simulink model "MMAE_laneChangeParametricWithMeasurements"  (R2018b)
settings: Solver=FixedStepAuto  StartTime=0.0  StopTime=15  FixedStep=1e-3  RelTol=1e-3
values from neighbouring files (symbols this model uses):
  A = obj.A    [LeftLaneChangeRelativeMotionModel.m]    (also in initialization.m = 1.75; laneChangeSinusoidalFcn.m = 1.75; laneChangeSinusoidalJacobianFcn.m = 1.75; leftLaneChangeParametricFcn.m = lateral_dist/2)
  Ts = 0.1    [KinematicBicycleModel.m]    (also in LeftLaneChangeSinusoidalMotionModel.m; LinearizedBicycleModel.m; SimplifiedKinematicBicycleModel.m; amm_rel_test.m)
  vx = X(2)    [cv_model_fun.m]    (also in initialization.m = 10)
  vy = X(4)    [cv_model_fun.m]    (also in initialization.m = 0)
  w = obj.w    [LeftLaneChangeRelativeMotionModel.m]    (also in ctra_model_fun.m = X(6); ctrv_model_fun.m = X(5); initialization.m = 0.0314159265359; laneChangeSinusoidalFcn.m = 0.0209439510239)
  x = X(1)    [KinematicBicycleModel.m]    (also in SimplifiedKinematicBicycleModel.m; behavior_model.m = 0:0.01:20; cca_model_fun.m; ctra_model_fun.m)
  y = X(2)    [KinematicBicycleModel.m]    (also in SimplifiedKinematicBicycleModel.m; behavior_model.m = [distances velocities]; cca_model_fun.m; ctra_model_fun.m)
  y_init = lanewidth/2    (= 1.75)    [initialization.m]    (also in laneChangeSinusoidalFcn.m; laneChangeSinusoidalJacobianFcn.m; leftLaneChangeSinusoidalFcn.m; leftLaneChangeSinusoidalJacobianFcn.m)
libraries: simulink x7
settings Model: Creator=jasprit  LastModifiedBy=jasprit
settings SFSimCC: SimUseLocalCustomCode=off
settings RTWCC: RTWUseLocalCustomCode=off

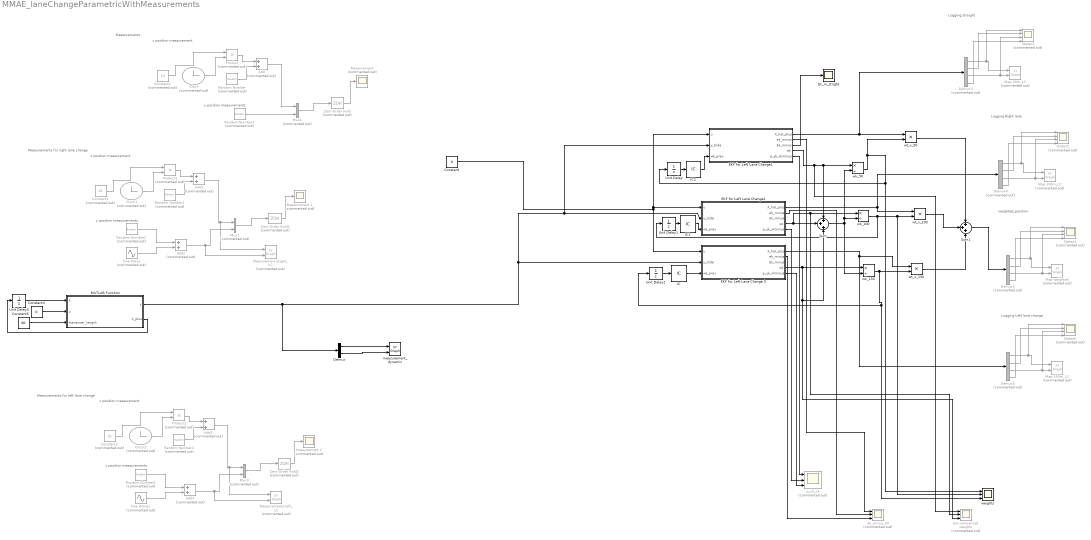
== system MMAE_laneChangeParametricWithMeasurements ==
  note: Logging Left lane change
  note: Logging straight
  note: Logging Right lane
  note: y position measurements
  note: x position measurement
  note: Measurements
  note: x position measurement
  note: Measurements for right lane change
  note: y position measurements
  note: y position measurements
  note: Measurements for left lane change
  note: x position measurement
  note: weighted_position
  Add{,1..4} (5 alike) : Sum  Commented=on
  Clock : Clock  Commented=on
  Clock1 : Clock  Commented=on
  Clock2 : Clock  Commented=on
  Constant : Constant  Value=0
  Constant1 : Constant  Commented=on  Value=10
  Constant2 : Constant  Commented=on  Value=10
  Constant3 : Constant  Commented=on  Value=10
  Constant4 : Constant  Value=0  SampleTime=Ts
  Constant5 : Constant  Value=60  SampleTime=Ts
  Demux : Demux  Outputs=2
  Demux{1,3..5} (4 alike) : Demux  Commented=on
  EKF for Left Lane Change 3 : Subsystem
  EKF for Left Lane Change1 : Subsystem
  EKF for Left Lane Change2 : Subsystem
  Ek_m_stright : Scope
  IC : InitialCondition  Value=1/3
  IC1 : InitialCondition  Value=1/3
  IC2 : InitialCondition  Value=1/3
  MATLAB Function : MATLAB Function  TreatAsAtomicUnit=on
  Map-100m_LC : simulink/Sinks/XY Graph  Commented=on  xmin=-1  xmax=200  ymin=-5  ymax=5  st=-1
  Map-150m_LC : simulink/Sinks/XY Graph  Commented=on  xmin=-1  xmax=200  ymin=-5  ymax=5  st=-1
  Map-50m_LC : simulink/Sinks/XY Graph  Commented=on  xmin=-1  xmax=200  ymin=-5  ymax=5  st=-1
  Map-weighted : simulink/Sinks/XY Graph  Commented=on  xmin=-1  xmax=200  ymin=-5  ymax=5  st=-1
  "Measurement " : Scope  Commented=on
  Measurement 1 : Scope  Commented=on
  Measurement 2 : Scope  Commented=on
  Measurement_Right_LC : simulink/Sinks/XY Graph  Commented=on  xmin=-1  xmax=200  ymin=-5  ymax=5  st=-1
  Measurements-left_LC : simulink/Sinks/XY Graph  Commented=on  xmin=-1  xmax=400  ymin=-5  ymax=5  st=-1
  Mux1 : Mux  Commented=on  Inputs=2
  Mux2 : Mux  Commented=on  Inputs=2
  Mux3 : Mux  Commented=on  Inputs=2
  Product : Product  Commented=on
  Product1 : Product  Commented=on
  Product2 : Product  Commented=on
  Random Number : RandomNumber  Commented=on  Variance=0.1  SampleTime=Ts
  Random Number1 : RandomNumber  Commented=on  Variance=0.1  SampleTime=Ts
  Random Number2 : RandomNumber  Commented=on  Variance=0.2  SampleTime=Ts
  Random Number3 : RandomNumber  Commented=on  Variance=0.2  SampleTime=Ts
  Random Number4 : RandomNumber  Commented=on  Variance=0.0025  SampleTime=Ts
  Random Number5 : RandomNumber  Commented=on  Variance=0.0025  SampleTime=Ts
  Sine Wave : Sin  Commented=on  Amplitude=A  Bias=-A  Frequency=w*vx  Phase=+pi/2  SampleTime=Ts
  Sine Wave1 : Sin  Commented=on  Amplitude=A  Bias=y_init  Frequency=w*vx  Phase=-pi/2  SampleTime=Ts
  States{1,4..6} (4 alike) : Scope  Commented=on  NumInputPorts=4
  Sum : Sum  Inputs=+++
  Sum1 : Sum  Inputs=+++
  Unit Delay : UnitDelay  SampleTime=-1
  Unit Delay1 : UnitDelay  SampleTime=-1
  Unit Delay2 : UnitDelay  SampleTime=-1
  Unit Delay3 : UnitDelay  InitialCondition=[x vx y vy]  SampleTime=Ts
  Zero-Order Hold : ZeroOrderHold  Commented=on  SampleTime=Ts
  Zero-Order Hold1 : ZeroOrderHold  Commented=on  SampleTime=Ts
  Zero-Order Hold2 : ZeroOrderHold  Commented=on  SampleTime=Ts
  ek_minus_All : Scope  Commented=on  NumInputPorts=3
  measurement_dynamic : simulink/Sinks/XY Graph  xmin=-1  xmax=200  ymin=-5  ymax=5  st=-1
  p_yk_xk : Scope  Commented=on  NumInputPorts=3
  pre-normalized weights : Scope  Commented=on  NumInputPorts=3
  weights : Scope  NumInputPorts=3
  wk_100 : Product  Inputs=*/
  wk_150 : Product  Inputs=*/
  wk_50 : Product  Inputs=*/
  wt_x_100 : Product  Inputs=**
  wt_x_150 : Product  Inputs=**
  wt_x_50 : Product  Inputs=**
  wires:
  Constant2/1 -> Product/1
  Clock/1 -> Product/2
  Product/1 -> Add/1
  Random Number/1 -> Add/2
  Add/1 -> Mux1/1
  Mux1/1 -> Zero-Order Hold/1
  Random Number3/1 -> Mux1/2
  Zero-Order Hold1/1 -> Measurement 1/1
  Product1/1 -> Add1/1
  Clock1/1 -> Product1/2
  Constant1/1 -> Product1/1
  Mux2/1 -> Zero-Order Hold1/1
  Add1/1 -> Measurement_Right_LC/1, Mux2/1
  Random Number1/1 -> Add1/2
  Random Number2/1 -> Add2/1
  Sine Wave/1 -> Add2/2
  Add2/1 -> Measurement_Right_LC/2, Mux2/2
  Random Number5/1 -> Add4/1
  Add3/1 -> Measurements-left_LC/1, Mux3/1
  Clock2/1 -> Product2/2
  Sine Wave1/1 -> Add4/2
  Product2/1 -> Add3/1
  Random Number4/1 -> Add3/2
  Constant3/1 -> Product2/1
  Mux3/1 -> Zero-Order Hold2/1
  Add4/1 -> Measurements-left_LC/2, Mux3/2
  Zero-Order Hold/1 -> "Measurement "/1
  Demux3/1 -> States4/1, Map-50m_LC/1
  Demux3/4 -> States4/4
  Demux3/2 -> States4/2
  Demux3/3 -> Map-50m_LC/2, States4/3
  Constant/1 -> EKF for Left Lane Change2/1(u), EKF for Left Lane Change1/1(u), EKF for Left Lane Change 3/1(u)
  Demux4/1 -> States5/1, Map-100m_LC/1
  Demux4/2 -> States5/2
  Demux4/4 -> States5/4
  Demux4/3 -> Map-100m_LC/2, States5/3
  Demux5/1 -> States6/1, Map-150m_LC/1
  Demux5/4 -> States6/4
  Demux5/3 -> Map-150m_LC/2, States6/3
  Demux5/2 -> States6/2
  EKF for Left Lane Change 3/1(X_hat_plus) -> wt_x_150/1, Demux5/1
  EKF for Left Lane Change2/1(X_hat_plus) -> Demux4/1, wt_x_100/1
  EKF for Left Lane Change 3/4(wk) -> wk_150/1, pre-normalized weights/3, Sum/3
  EKF for Left Lane Change2/4(wk) -> pre-normalized weights/2, wk_100/1, Sum/2
  Sum/1 -> wk_150/2, wk_50/2, wk_100/2
  wk_50/1 -> Unit Delay/1, weights/1, wt_x_50/2
  wk_100/1 -> Unit Delay1/1, weights/2, wt_x_100/2
  wk_150/1 -> Unit Delay2/1, weights/3, wt_x_150/2
  wt_x_100/1 -> Sum1/2
  wt_x_50/1 -> Sum1/1
  wt_x_150/1 -> Sum1/3
  Demux1/1 -> States1/1, Map-weighted/1
  Demux1/4 -> States1/4
  Demux1/2 -> States1/2
  Demux1/3 -> States1/3, Map-weighted/2
  Sum1/1 -> Demux1/1
  IC2/1 -> EKF for Left Lane Change1/3(wk_prev)
  Unit Delay/1 -> IC2/1
  IC1/1 -> EKF for Left Lane Change2/3(wk_prev)
  Unit Delay1/1 -> IC1/1
  IC/1 -> EKF for Left Lane Change 3/3(wk_prev)
  Unit Delay2/1 -> IC/1
  EKF for Left Lane Change2/2(ek_minus) -> ek_minus_All/2
  EKF for Left Lane Change 3/2(ek_minus) -> ek_minus_All/3
  MATLAB Function/1(y) -> EKF for Left Lane Change 3/2(y_tilde), EKF for Left Lane Change1/2(y_tilde), EKF for Left Lane Change2/2(y_tilde), Demux/1
  Zero-Order Hold2/1 -> Measurement 2/1
  EKF for Left Lane Change2/5(p_yk_xkminus) -> p_yk_xk/2
  EKF for Left Lane Change 3/5(p_yk_xkminus) -> p_yk_xk/3
  EKF for Left Lane Change1/1(X_hat_plus) -> Demux3/1, wt_x_50/1
  EKF for Left Lane Change1/2(ek_minus) -> ek_minus_All/1
  EKF for Left Lane Change1/4(wk) -> pre-normalized weights/1, wk_50/1, Sum/1
  EKF for Left Lane Change1/5(p_yk_xkminus) -> p_yk_xk/1
  EKF for Left Lane Change1/3(Ek_minus) -> Ek_m_stright/1
  Unit Delay3/1 -> MATLAB Function/1(X)
  MATLAB Function/2(X_plus) -> Unit Delay3/1
  Constant4/1 -> MATLAB Function/2(u)
  Demux/1 -> measurement_dynamic/1
  Demux/2 -> measurement_dynamic/2
  Constant5/1 -> MATLAB Function/3(maneuver_length)

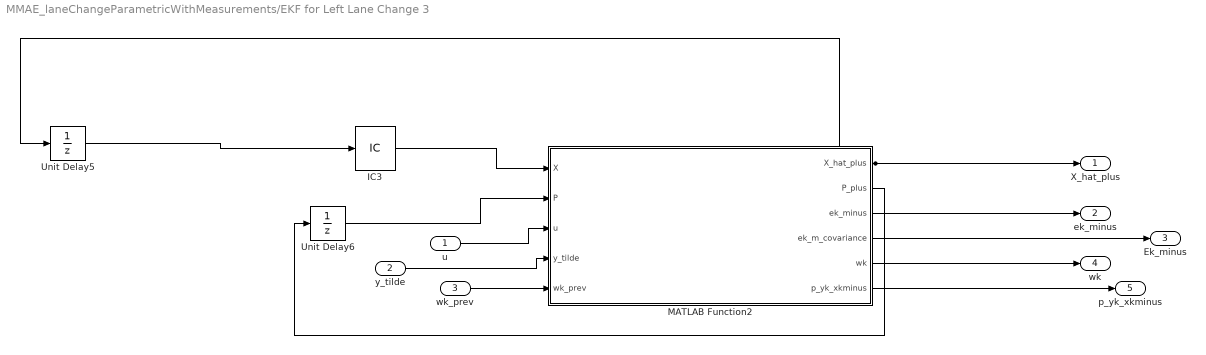
== system MMAE_laneChangeParametricWithMeasurements/EKF for Left Lane Change 3 ==
  u : Inport
  y_tilde : Inport  Port=2
  wk_prev : Inport  Port=3
  IC3 : InitialCondition  Value=[x vx y vy]
  MATLAB Function2 : MATLAB Function  TreatAsAtomicUnit=on
  Unit Delay5 : UnitDelay  SampleTime=-1
  Unit Delay6 : UnitDelay  SampleTime=-1
  X_hat_plus : Outport
  ek_minus : Outport  Port=2
  Ek_minus : Outport  Port=3
  wk : Outport  Port=4
  p_yk_xkminus : Outport  Port=5
  wires:
  MATLAB Function2/2(P_plus) -> Unit Delay6/1
  u/1 -> MATLAB Function2/3(u)
  Unit Delay5/1 -> IC3/1
  y_tilde/1 -> MATLAB Function2/4(y_tilde)
  MATLAB Function2/1(X_hat_plus) -> X_hat_plus/1, Unit Delay5/1
  IC3/1 -> MATLAB Function2/1(X)
  Unit Delay6/1 -> MATLAB Function2/2(P)
  MATLAB Function2/3(ek_minus) -> ek_minus/1
  MATLAB Function2/4(ek_m_covariance) -> Ek_minus/1
  MATLAB Function2/5(wk) -> wk/1
  MATLAB Function2/6(p_yk_xkminus) -> p_yk_xkminus/1
  wk_prev/1 -> MATLAB Function2/5(wk_prev)

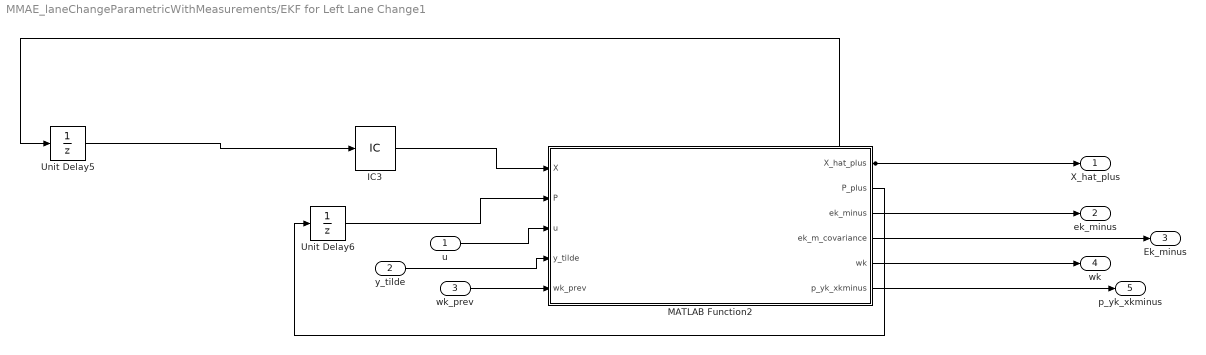
== system MMAE_laneChangeParametricWithMeasurements/EKF for Left Lane Change1 ==
  u : Inport
  y_tilde : Inport  Port=2
  wk_prev : Inport  Port=3
  IC3 : InitialCondition  Value=[x vx y vy]
  MATLAB Function2 : MATLAB Function  TreatAsAtomicUnit=on
  Unit Delay5 : UnitDelay  SampleTime=-1
  Unit Delay6 : UnitDelay  SampleTime=-1
  X_hat_plus : Outport
  ek_minus : Outport  Port=2
  Ek_minus : Outport  Port=3
  wk : Outport  Port=4
  p_yk_xkminus : Outport  Port=5
  wires:
  MATLAB Function2/2(P_plus) -> Unit Delay6/1
  u/1 -> MATLAB Function2/3(u)
  Unit Delay5/1 -> IC3/1
  y_tilde/1 -> MATLAB Function2/4(y_tilde)
  MATLAB Function2/1(X_hat_plus) -> X_hat_plus/1, Unit Delay5/1
  IC3/1 -> MATLAB Function2/1(X)
  Unit Delay6/1 -> MATLAB Function2/2(P)
  MATLAB Function2/3(ek_minus) -> ek_minus/1
  MATLAB Function2/4(ek_m_covariance) -> Ek_minus/1
  MATLAB Function2/5(wk) -> wk/1
  MATLAB Function2/6(p_yk_xkminus) -> p_yk_xkminus/1
  wk_prev/1 -> MATLAB Function2/5(wk_prev)

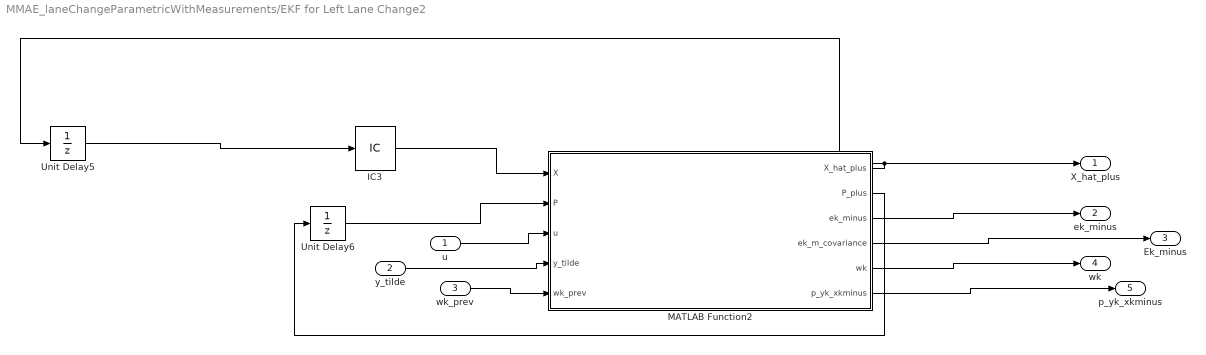
== system MMAE_laneChangeParametricWithMeasurements/EKF for Left Lane Change2 ==
  u : Inport
  y_tilde : Inport  Port=2
  wk_prev : Inport  Port=3
  IC3 : InitialCondition  Value=[x vx y vy]
  MATLAB Function2 : MATLAB Function  TreatAsAtomicUnit=on
  Unit Delay5 : UnitDelay  SampleTime=-1
  Unit Delay6 : UnitDelay  SampleTime=-1
  X_hat_plus : Outport
  ek_minus : Outport  Port=2
  Ek_minus : Outport  Port=3
  wk : Outport  Port=4
  p_yk_xkminus : Outport  Port=5
  wires:
  MATLAB Function2/2(P_plus) -> Unit Delay6/1
  u/1 -> MATLAB Function2/3(u)
  Unit Delay5/1 -> IC3/1
  y_tilde/1 -> MATLAB Function2/4(y_tilde)
  MATLAB Function2/1(X_hat_plus) -> Unit Delay5/1, X_hat_plus/1
  IC3/1 -> MATLAB Function2/1(X)
  Unit Delay6/1 -> MATLAB Function2/2(P)
  MATLAB Function2/3(ek_minus) -> ek_minus/1
  MATLAB Function2/4(ek_m_covariance) -> Ek_minus/1
  MATLAB Function2/5(wk) -> wk/1
  MATLAB Function2/6(p_yk_xkminus) -> p_yk_xkminus/1
  wk_prev/1 -> MATLAB Function2/5(wk_prev)

== matlab function MMAE_laneChangeParametricWithMeasurements/EKF for Left Lane Change2/MATLAB Function2 ==
  data: X input; P input; u input; X_hat_plus output; y_tilde input; P_plus output; ek_minus output; ek_m_covariance output; wk output; p_yk_xkminus output; wk_prev input
function [X_hat_plus, P_plus, ek_minus, ek_m_covariance, wk, p_yk_xkminus] = EKFLeftLaneChangeCustom(X, P, u, y_tilde, wk_prev)

    maneuver_length = 100;  %meters
    lane_center_to_center_distance = 3.5;   %meters
    
    %%
    %TODO: See how can this be moved out of the function later
    %sampling time
    Ts = 0.01;

    % measurement noise covariance
%     R = [0.2 0; 0 0.2];
    R = [0.0025 0; 0 0.0025];
    
    % process noise covariance
%     Q = diag([0.5 5.0 0.5 5.0]);
    Q = diag([0.001 0.001 0.001 0.001]);

    % states - X = [x vx y vy] -     
    Ck = [1 0 0 0; 0 0 1 0];

    F = leftLaneChangeParametricJacobianFcn(X, u, maneuver_length, lane_center_to_center_distance);
    %%
    % Now estimate states using kalman filter
    
    %predict
    xhat_minus = leftLaneChangeParametricFcn(X, u, maneuver_length, lane_center_to_center_distance);
    P_minus = (F * P * F') + Ts*Q;
    yhat_minus = Ck * xhat_minus;

    %correct
    ek_minus = y_tilde - yhat_minus;    %residual
    ek_m_covariance = Ck * P_minus *Ck' + R;    %residual covariance
    K = P_minus * Ck' * inv(ek_m_covariance);
    X_hat_plus = xhat_minus + K * ek_minus;
    P_plus = (eye(4) - K * Ck) * P_minus;
    
    %calculate MMAE weights
    p_yk_xkminus = 1/sqrt(det(2*pi*ek_m_covariance))*exp(-1/2 * ek_minus'* inv(ek_m_covariance) * ek_minus);
    wk = wk_prev * p_yk_xkminus;

    
end

== matlab function MMAE_laneChangeParametricWithMeasurements/EKF for Left Lane Change1/MATLAB Function2 ==
  data: X input; P input; u input; X_hat_plus output; y_tilde input; P_plus output; ek_minus output; ek_m_covariance output; wk output; p_yk_xkminus output; wk_prev input
function [X_hat_plus, P_plus, ek_minus, ek_m_covariance, wk, p_yk_xkminus] = EKFLeftLaneChangeCustom(X, P, u, y_tilde, wk_prev)

    maneuver_length = 50;  %meters
    lane_center_to_center_distance = 3.5;   %meters
    
    %%
    %TODO: See how can this be moved out of the function later
    %sampling time
    Ts = 0.01;

    % measurement noise covariance
%     R = [0.2 0; 0 0.2];
    R = [0.0025 0; 0 0.0025];
    
    % process noise covariance
%     Q = diag([0.5 5.0 0.5 5.0]);
    Q = diag([0.001 0.001 0.001 0.001]);

    % states - X = [x vx y vy] -     
    Ck = [1 0 0 0; 0 0 1 0];

    F = leftLaneChangeParametricJacobianFcn(X, u, maneuver_length, lane_center_to_center_distance);
    %%
    % Now estimate states using kalman filter
    
    %predict
    xhat_minus = leftLaneChangeParametricFcn(X, u, maneuver_length, lane_center_to_center_distance);
    P_minus = (F * P * F') + Ts*Q;
    yhat_minus = Ck * xhat_minus;

    %correct
    ek_minus = y_tilde - yhat_minus;    %residual
    ek_m_covariance = Ck * P_minus *Ck' + R;    %residual covariance
    K = P_minus * Ck' * inv(ek_m_covariance);
    X_hat_plus = xhat_minus + K * ek_minus;
    P_plus = (eye(4) - K * Ck) * P_minus;
    
    %calculate MMAE weights
    p_yk_xkminus = 1/sqrt(det(2*pi*ek_m_covariance))*exp(-1/2 * ek_minus'* inv(ek_m_covariance) * ek_minus);
    wk = wk_prev * p_yk_xkminus;

    
end

== matlab function MMAE_laneChangeParametricWithMeasurements/EKF for Left Lane Change 3/MATLAB Function2 ==
  data: X input; P input; u input; X_hat_plus output; y_tilde input; P_plus output; ek_minus output; ek_m_covariance output; wk output; p_yk_xkminus output; wk_prev input
function [X_hat_plus, P_plus, ek_minus, ek_m_covariance, wk, p_yk_xkminus] = EKFLeftLaneChangeCustom(X, P, u, y_tilde, wk_prev)

    maneuver_length = 150;  %meters
    lane_center_to_center_distance = 3.5;   %meters
    
    %%
    %TODO: See how can this be moved out of the function later
    %sampling time
    Ts = 0.01;

    % measurement noise covariance
%     R = [0.2 0; 0 0.2];
    R = [0.0025 0; 0 0.0025];
    
    % process noise covariance
%     Q = diag([0.5 5.0 0.5 5.0]);
    Q = diag([0.001 0.001 0.001 0.001]);

    % states - X = [x vx y vy] -     
    Ck = [1 0 0 0; 0 0 1 0];

    F = leftLaneChangeParametricJacobianFcn(X, u, maneuver_length, lane_center_to_center_distance);
    %%
    % Now estimate states using kalman filter
    
    %predict
    xhat_minus = leftLaneChangeParametricFcn(X, u, maneuver_length, lane_center_to_center_distance);
    P_minus = (F * P * F') + Ts*Q;
    yhat_minus = Ck * xhat_minus;

    %correct
    ek_minus = y_tilde - yhat_minus;    %residual
    ek_m_covariance = Ck * P_minus *Ck' + R;    %residual covariance
    K = P_minus * Ck' * inv(ek_m_covariance);
    X_hat_plus = xhat_minus + K * ek_minus;
    P_plus = (eye(4) - K * Ck) * P_minus;
    
    %calculate MMAE weights
    p_yk_xkminus = 1/sqrt(det(2*pi*ek_m_covariance))*exp(-1/2 * ek_minus'* inv(ek_m_covariance) * ek_minus);
    wk = wk_prev * p_yk_xkminus;

    
end

== matlab function MMAE_laneChangeParametricWithMeasurements/MATLAB Function ==
  data: X input; u input; y output; X_plus output; maneuver_length input
function [y, X_plus]= measurementsForLaneChange(X, u, maneuver_length)

    Ts = 0.01;
%     maneuver_length = 150;  %m
    lane_center_to_center_distance = 3.5;   %meters

    % states - X = [x vx y vy] -     
    Ck = [1 0 0 0; 0 0 1 0];

    % measurement noise std_dev
    R_sigma = [0.05 0; 0 0.05];
    
    % process noise std dev
    sigma_matrix = diag([0.032 0.032 0.032 0.032]);
    
    X_plus = leftLaneChangeParametricFcn(X, u, maneuver_length, lane_center_to_center_distance) + sqrt(Ts)*sigma_matrix*randn(4,1);

    y = Ck * X_plus + R_sigma * randn(2,1);
    
end
